simulink model "gps_simulation"  (R2021a)
settings: Solver=VariableStepAuto  StartTime=0.0  StopTime=10.0  RelTol=1e-3
libraries: simulink x5
settings Model: Creator=avall  LastModifiedBy=avall

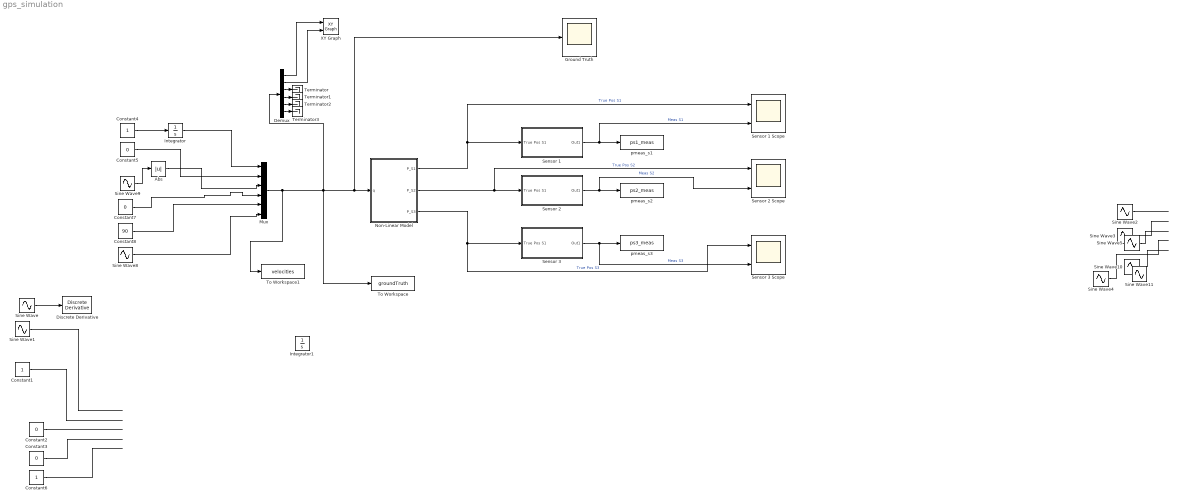
== system gps_simulation ==
  Abs : Abs
  Constant1 : Constant
  Constant{2..3,5,7} (4 alike) : Constant  Value=0
  Constant4 : Constant
  Constant6 : Constant
  Constant8 : Constant  Value=90
  Demux : Demux  Outputs=6
  Discrete Derivative : simulink/Discrete/Discrete Derivative  gainval=1.0  ICPrevScaledInput=0.0  OutMin=[]  OutMax=[]  OutDataType=fixdt(1, 16)  OutScaling=2^-10  DoSatur=off
  Ground Truth : Scope
  Integrator : Integrator
  Integrator1 : Integrator
  Mux : Mux  Inputs=6
  "Non-Linear Model " : Subsystem
  Sensor 1 : Subsystem
  Sensor 1 Scope : Scope  NumInputPorts=2
  Sensor 2 : Subsystem
  Sensor 2 Scope : Scope  NumInputPorts=2
  Sensor 3 : Subsystem
  Sensor 3 Scope : Scope  NumInputPorts=2
  Sine Wave{,1,4,8..11} (7 alike) : Sin  SampleTime=0.1
  Sine Wave2 : Sin  Amplitude=2  SampleTime=0.1
  Sine Wave3 : Sin  Amplitude=2  SampleTime=0.1
  Sine Wave5 : Sin  Amplitude=2  SampleTime=0.1
  Terminator{,1..3} (4 alike) : Terminator
  To Workspace : ToWorkspace  VariableName=groundTruth  SaveFormat=Structure With Time  SampleTime=0.1
  To Workspace1 : ToWorkspace  VariableName=velocities  SaveFormat=Structure With Time  SampleTime=0.1
  XY Graph : simulink/Sinks/XY Graph  xmin=-1  xmax=1  ymin=-1  ymax=3  st=-1
  pmeas_s1 : ToWorkspace  VariableName=ps1_meas  SampleTime=-1
  pmeas_s2 : ToWorkspace  VariableName=ps2_meas  SampleTime=-1
  pmeas_s3 : ToWorkspace  VariableName=ps3_meas  SampleTime=-1
  wires:
  Sensor 1/1(Out1) -> Sensor 1 Scope/2, pmeas_s1/1  "Meas S1"
  "Non-Linear Model "/1(P_S1) -> Sensor 1 Scope/1, Sensor 1/1(True Pos S1)  "True Pos S1"
  Sensor 2/1(Out1) -> Sensor 2 Scope/2, pmeas_s2/1  "Meas S2"
  "Non-Linear Model "/2(P_S2) -> Sensor 2/1(True Pos S1), Sensor 2 Scope/1  "True Pos S2"
  Sensor 3/1(Out1) -> Sensor 3 Scope/2, pmeas_s3/1  "Meas S3"
  "Non-Linear Model "/3(P_S3) -> Sensor 3/1(True Pos S1), Sensor 3 Scope/1  "True Pos S3"
  Demux/1 -> XY Graph/1
  Demux/2 -> XY Graph/2
  Demux/3 -> Terminator/1
  Demux/4 -> Terminator1/1
  Demux/5 -> Terminator2/1
  Demux/6 -> Terminator3/1
  Sine Wave2/1 -> ?
  Sine Wave3/1 -> ?
  Sine Wave5/1 -> ?
  Sine Wave4/1 -> ?
  Sine Wave10/1 -> ?
  Constant4/1 -> Integrator/1
  Constant7/1 -> Mux/4
  Abs/1 -> Mux/3
  Sine Wave9/1 -> Abs/1
  Constant5/1 -> Mux/2
  Constant8/1 -> Mux/5
  Sine Wave8/1 -> Mux/6
  Mux/1 -> Ground Truth/1, "Non-Linear Model "/1(q), Demux/1, To Workspace/1, To Workspace1/1
  Sine Wave/1 -> Discrete Derivative/1
  Constant2/1 -> ?
  Constant6/1 -> ?
  Constant1/1 -> ?
  Sine Wave1/1 -> ?
  Constant3/1 -> ?
  Integrator/1 -> Mux/1

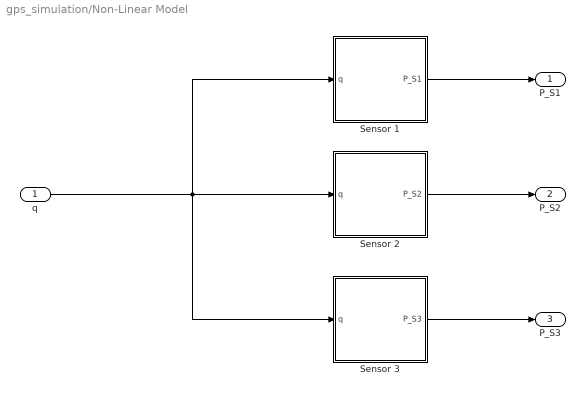
== system gps_simulation/Non-Linear Model  ==
  q : Inport
  Sensor 1 : MATLAB Function  TreatAsAtomicUnit=on
  Sensor 2 : MATLAB Function  TreatAsAtomicUnit=on
  Sensor 3 : MATLAB Function  TreatAsAtomicUnit=on
  P_S1 : Outport
  P_S2 : Outport  Port=2
  P_S3 : Outport  Port=3
  wires:
  q/1 -> Sensor 3/1(q), Sensor 2/1(q), Sensor 1/1(q)
  Sensor 3/1(P_S3) -> P_S3/1
  Sensor 2/1(P_S2) -> P_S2/1
  Sensor 1/1(P_S1) -> P_S1/1

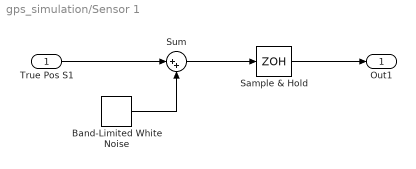
== system gps_simulation/Sensor 1 ==
  True Pos S1 : Inport
  Band-Limited White Noise : simulink/Sources/Band-Limited White Noise  Cov=(0.01)^2  Ts=0.1  seed=[23341]
  Sample & Hold : ZeroOrderHold  SampleTime=0.1
  Sum : Sum  Inputs=|++
  Out1 : Outport
  wires:
  Sample & Hold/1 -> Out1/1
  True Pos S1/1 -> Sum/1
  Band-Limited White Noise/1 -> Sum/2
  Sum/1 -> Sample & Hold/1

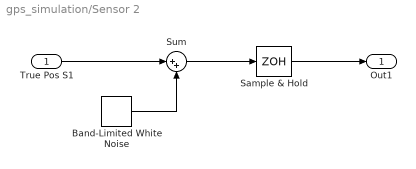
== system gps_simulation/Sensor 2 ==
  True Pos S1 : Inport
  Band-Limited White Noise : simulink/Sources/Band-Limited White Noise  Cov=(0.01)^2  Ts=0.1  seed=[23341]
  Sample & Hold : ZeroOrderHold  SampleTime=0.1
  Sum : Sum  Inputs=|++
  Out1 : Outport
  wires:
  Sample & Hold/1 -> Out1/1
  True Pos S1/1 -> Sum/1
  Band-Limited White Noise/1 -> Sum/2
  Sum/1 -> Sample & Hold/1

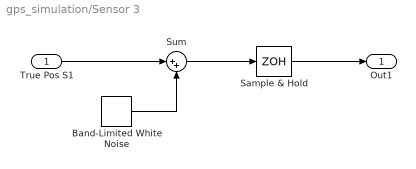
== system gps_simulation/Sensor 3 ==
  True Pos S1 : Inport
  Band-Limited White Noise : simulink/Sources/Band-Limited White Noise  Cov=(0.01)^2  Ts=0.1  seed=[23341]
  Sample & Hold : ZeroOrderHold  SampleTime=0.1
  Sum : Sum  Inputs=|++
  Out1 : Outport
  wires:
  Sample & Hold/1 -> Out1/1
  True Pos S1/1 -> Sum/1
  Band-Limited White Noise/1 -> Sum/2
  Sum/1 -> Sample & Hold/1

== matlab function gps_simulation/Non-Linear Model /Sensor 2 ==
  data: q input; P_S2 output
function P_S2 = pos_s2(q)
%UPDATE_HS2
%    H_S2 = UPDATE_HS2(X,Y,Z,DX,DY,DZ,DDX,DDY,DDZ,RX,RY,RZ,DRX,DRY,DRZ,DDRX,DDRY,DDRZ,L,DT)

%    This function was generated by the Symbolic Math Toolbox version 8.7.
%    20-Oct-2021 23:21:27
L = 0.5; 
x = q(1);
y = q(2);
z = q(3);
rx = q(4);
ry = q(5);
rz = q(6);

t2 = cos(rx);
t3 = cos(rz);
t4 = sin(rx);
t5 = sin(ry);
t6 = sin(rz);
P_S2 = [x+L.*(t2.*t6-t3.*t4.*t5);y-L.*(t2.*t3+t4.*t5.*t6);z-L.*t4.*cos(ry)];

== matlab function gps_simulation/Non-Linear Model /Sensor 1 ==
  data: q input; P_S1 output
function P_S1 = pos_s1(q)
%UPDATE_HS1
%    H_S1 = UPDATE_HS1(X,Y,Z,DX,DY,DZ,DDX,DDY,DDZ,RX,RY,RZ,DRX,DRY,DRZ,DDRX,DDRY,DDRZ,L,DT)

%    This function was generated by the Symbolic Math Toolbox version 8.7.
%    20-Oct-2021 23:21:27
L = 0.5; 
x = q(1);
y = q(2);
z = q(3);
rx = q(4);
ry = q(5);
rz = q(6);

t2 = cos(rx);
t3 = cos(rz);
t4 = sin(rx);
t5 = sin(ry);
t6 = sin(rz);
P_S1 = [x-L.*(t2.*t6-t3.*t4.*t5);y+L.*(t2.*t3+t4.*t5.*t6);z+L.*t4.*cos(ry)];

== matlab function gps_simulation/Non-Linear Model /Sensor 3 ==
  data: q input; P_S3 output
function P_S3 = pos_s3(q)
%UPDATE_HS3
%    H_S3 = UPDATE_HS3(X,Y,Z,DX,DY,DZ,DDX,DDY,DDZ,RX,RY,RZ,DRX,DRY,DRZ,DDRX,DDRY,DDRZ,L,DT)

%    This function was generated by the Symbolic Math Toolbox version 8.7.
%    20-Oct-2021 23:21:28
L = 0.5; 
x = q(1);
y = q(2);
z = q(3);
rx = q(4);
ry = q(5);
rz = q(6);

t2 = cos(ry);
P_S3 = [x+L.*t2.*cos(rz);y+L.*t2.*sin(rz);z-L.*sin(ry)];
